simulink model "TTypeInverter_R2022a"  (R2022a)
settings: Solver=ode23t  StartTime=0.0  StopTime=0.2  RelTol=1e-3  EnableMultiTasking=on
values from neighbouring files (symbols this model uses):
  C_c = 30*10^-6    (= 3e-05)    [TTypeInverterVals.m]
  den = abs(G_pr_r_z.Denominator{1,1})    [TTypeInverterVals.m]
  den15 = abs(G_pr_r_15_z.Denominator{1,1})    [TTypeInverterVals.m]
  den21 = abs(G_pr_r_21_z.Denominator{1,1})    [TTypeInverterVals.m]
  den5 = abs(G_pr_r_5_z.Denominator{1,1})    [TTypeInverterVals.m]
  den7 = abs(G_pr_r_7_z.Denominator{1,1})    [TTypeInverterVals.m]
  f_o = 50    [TTypeInverterVals.m]
  G_diff_z = c2d(G_diff_s,Ts,opt)    [ControllerDesign.m]    (also in TTypeInverterVals.m = c2d(G_diff_s,Ts,'foh'))
  Kc = 2.5    [ControllerDesign.m]    (also in TTypeInverterVals.m)
  Klim = 5    [TTypeInverterVals.m]
  Kp = 1/mag/(10^(1.14/20))    [ControllerDesign.m]    (also in TTypeInverterVals.m = 0.9444)
  Kr = omega_c_o/2    (= 3141.59265359)    [ControllerDesign.m]    (also in TTypeInverterVals.m)
  N = 26    [Inductance.m]    (also in TTypeInverterVals.m = [0])
  num = abs(G_pr_r_z.Numerator{1,1})    [TTypeInverterVals.m]
  num15 = abs(G_pr_r_15_z.Numerator{1,1})    [TTypeInverterVals.m]
  num21 = abs(G_pr_r_21_z.Numerator{1,1})    [TTypeInverterVals.m]
  num5 = abs(G_pr_r_5_z.Numerator{1,1})    [TTypeInverterVals.m]
  num7 = abs(G_pr_r_7_z.Numerator{1,1})    [TTypeInverterVals.m]
  omega_o = fo*2*pi    (= 314.159265359)    [ControllerDesign.m]    (also in TTypeInverterVals.m)
  omega_w = 0.1*2*pi    (= 0.628318530718)    [ControllerDesign.m]    (also in TTypeInverterVals.m)
  pr_sat_val = ceil(3*io_nom)    [TTypeInverterVals.m]
  Q = eye(3)    [TTypeInverterVals.m]
  R = [R_iL 0 ... (first row only)    [TTypeInverterVals.m]
  R_l_20p = Vout^2/P_lin_20p    (= 10.58)    [TTypeInverterVals.m]
  R_l_3p = Vout/(P_max_3p/(Vout*3))    (= 2.116)    [TTypeInverterVals.m]
  R_l_80p = Vout^2/P_lin_80p    (= 2.645)    [TTypeInverterVals.m]
  R_l_nl = Vout^2/P_lin    (= 3.11176470588)    [TTypeInverterVals.m]
  R_l_nl_3p = Vout_3p^2/P_lin_3p    [TTypeInverterVals.m]
  R_Lc = 5.6e-3    (= 0.0056)    [TTypeInverterVals.m]
  R_nl_load = Uc^2/(0.66*S_tot)    (= 14.9121893939)    [TTypeInverterVals.m]
  R_nl_load_3p = Uc_3p^2/(0.66*S_tot_3p)    (= 4.97072979798)    [TTypeInverterVals.m]
  R_nl_s = 0.04*Vout^2/S_tot    (= 0.2645)    [TTypeInverterVals.m]
  R_nl_s_3p = 0.04*Vout_3p^2/S_tot_3p    [TTypeInverterVals.m]
  T_sw = 1/f_sw    (= 4.16666666667e-05)    [TTypeInverterVals.m]
  Tcomp = Ts/4    (= 2.60400009204e-06)    [TTypeInverterVals.m]
  Ts = 1/fs    (= 1.04166666667e-05)    [ControllerDesign.m]    (also in KalmanFilter.m = 2.08333333333e-05; TTypeInverterVals.m = 1.04160003681e-05)
  VDC = 800    [TTypeInverterVals.m]
  Vout_amp = Vout*sqrt(2)    [TTypeInverterVals.m]
undefined symbols (not defined in the file or in its folder): a0, a1, b0, b1, Discrete, G_ll_z, Ki, Kpc, KT, kv, Time, UKF_data
libraries: ee_lib x94, nesl_utility x48, fl_lib x39, dspstat3 x15, spsTriangleGeneratorLib x6, ctrlSharedLib x3, spsRMSLib x3, spsTHDLib x3
(part 3 of 5)

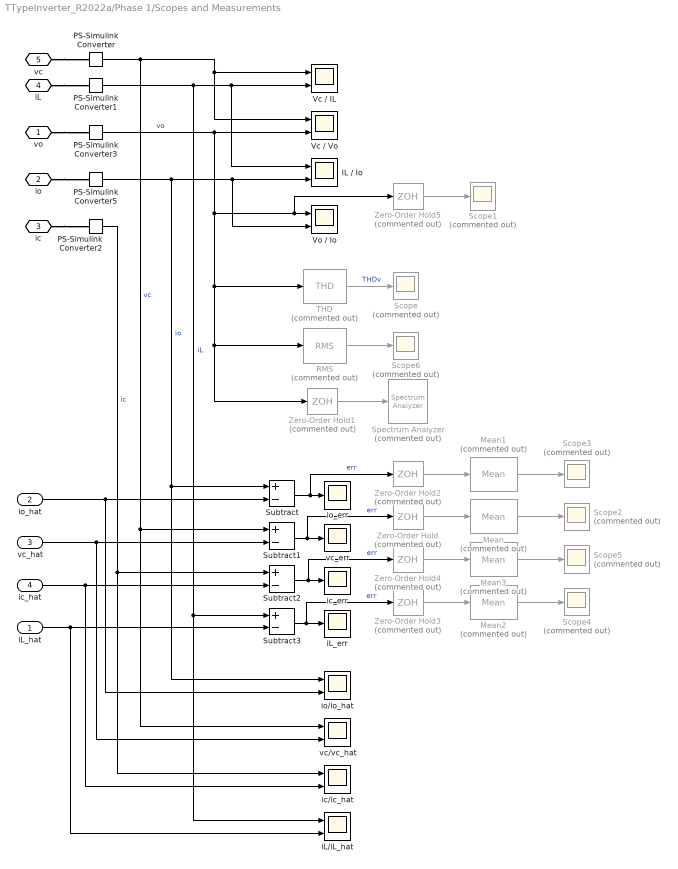
== system TTypeInverter_R2022a/Phase 1/Scopes and Measurements ==
  iL_hat : Inport
  io_hat : Inport  Port=2
  vc_hat : Inport  Port=3
  ic_hat : Inport  Port=4
  IL / Io : Scope  NumInputPorts=2
  Mean{,1..3} (4 alike) : dspstat3/Mean  Commented=on  run=on  InputProcessing=Columns as channels (frame based)  reset_popup=None  directionMode=Each column  dimension=1  roiEnable=off  roiType=Rectangles  roiPortion=Entire ROI  roiOutput=Individual statistics for each ROI  roiFlag=off  roundingMode=Floor  overflowMode=off  outputDataTypeStr=Inherit: Same as accumulator  outputMin=[]  outputMax=[]  outputLastDataTypeStr=Inherit: Same as accumulator
  PS-Simulink Converter{,1..3,5} (5 alike) : nesl_utility/PS-Simulink Converter  PhysicalDomain=network_engine_domain  SubClassName=ps_output  LeftPortType=input  RightPortType=output  PseudoPeriodic=off  Frequencies=[]  VectorFormat=inherit  Unit=inherit  AffineConversion=off
      settings: SourceProductBaseCode=SS,PW,VE
  RMS : spsRMSLib/RMS  Commented=on  TrueRMS=on  Freq=100  RMSInit=230  Ts=0
  Scope{,1..6} (7 alike) : Scope  Commented=on
  Spectrum Analyzer : SpectrumAnalyzer  Commented=on
  Subtract{,1..3} (4 alike) : Sum  Inputs=+-
  THD : spsTHDLib/THD  Commented=on  Freq=50  Ts=0
      settings: SourceProductBaseCode=PS
  Vc / IL : Scope  NumInputPorts=2
  Vc / Vo : Scope  NumInputPorts=2
  Vo / Io : Scope  NumInputPorts=2
  Zero-Order Hold{,2..4} (4 alike) : ZeroOrderHold  Commented=on  SampleTime=Ts/10
  Zero-Order Hold1 : ZeroOrderHold  Commented=on  SampleTime=1/100000
  Zero-Order Hold5 : ZeroOrderHold  Commented=on  SampleTime=T_sw/500
  iL/iL_hat : Scope  NumInputPorts=2
  iL_err : Scope
  ic/ic_hat : Scope  NumInputPorts=2
  ic_err : Scope
  io/io_hat : Scope  NumInputPorts=2
  io_err : Scope
  vc/vc_hat : Scope  NumInputPorts=2
  vc_err : Scope
  vo : PMIOPort  Side=Left
  io : PMIOPort  Port=2  Side=Left
  ic : PMIOPort  Port=3  Side=Left
  iL : PMIOPort  Port=4  Side=Left
  vc : PMIOPort  Port=5  Side=Left
  wires:
  PS-Simulink Converter1/1 -> iL/iL_hat/1, Subtract3/1, IL / Io/1, Vc / IL/2  "iL"
  PS-Simulink Converter/1 -> vc/vc_hat/1, Subtract1/1, Vc / Vo/1, Vc / IL/1  "vc"
  THD/1 -> Scope/1  "THDv"
  PS-Simulink Converter5/1 -> io/io_hat/1, Subtract/1, Vo / Io/2, IL / Io/2  "io"
  PS-Simulink Converter3/1 -> Vc / Vo/2, Zero-Order Hold5/1, Vo / Io/1, THD/1, RMS/1, Zero-Order Hold1/1  "vo"
  Zero-Order Hold1/1 -> Spectrum Analyzer/1
  io_hat/1 -> io/io_hat/2, Subtract/2
  Subtract/1 -> Zero-Order Hold2/1, io_err/1  "err"
  ic_hat/1 -> ic/ic_hat/2, Subtract2/2
  vc_hat/1 -> vc/vc_hat/2, Subtract1/2
  Subtract1/1 -> Zero-Order Hold/1, vc_err/1  "err"
  PS-Simulink Converter2/1 -> ic/ic_hat/1, Subtract2/1  "ic"
  Subtract2/1 -> Zero-Order Hold4/1, ic_err/1  "err"
  Mean/1 -> Scope2/1
  Zero-Order Hold/1 -> Mean/1
  Mean1/1 -> Scope3/1
  Zero-Order Hold2/1 -> Mean1/1
  iL_hat/1 -> iL/iL_hat/2, Subtract3/2
  Subtract3/1 -> Zero-Order Hold3/1, iL_err/1  "err"
  Mean2/1 -> Scope4/1
  Zero-Order Hold3/1 -> Mean2/1
  Mean3/1 -> Scope5/1
  Zero-Order Hold4/1 -> Mean3/1
  RMS/1 -> Scope6/1
  Zero-Order Hold5/1 -> Scope1/1
  connections:
  vc/RConn1 -- PS-Simulink Converter/LConn1
  iL/RConn1 -- PS-Simulink Converter1/LConn1
  vo/RConn1 -- PS-Simulink Converter3/LConn1
  io/RConn1 -- PS-Simulink Converter5/LConn1
  ic/RConn1 -- PS-Simulink Converter2/LConn1

== system TTypeInverter_R2022a/Phase 2/Controllers ==
  note: Voltage feedforward
  note: Current feedforward
  iL : Inport
  io_hat : Inport  Port=2
  vc : Inport  Port=3
  ic_hat : Inport  Port=4
  Current Controller : Subsystem
  Error Scope : Scope  NumInputPorts=2
  Gain : Gain  Gain=2/VDC
  Gain1 : Gain  Gain=R_Lc
  Reference Scope : Scope  NumInputPorts=2
  Saturation : Saturate  UpperLimit=VDC/2  LowerLimit=-VDC/2
  Sine Wave : Sin  Amplitude=Vout_amp  Frequency=f_o*2*pi  Phase=120*pi/180  SampleTime=Ts
  Sum : Sum  Inputs=|+-
  Sum1 : Sum  Inputs=++|
  Sum2 : Sum  Inputs=+++
  Sum3 : Sum  Inputs=-+|
  Transport Delay : TransportDelay  DelayTime=Tcomp
  Voltage Controller : Subsystem
  m : Outport
  vi_ref : Outport  Port=2
  wires:
  Transport Delay/1 -> m/1
  Voltage Controller/1(Out) -> Sum1/2, Reference Scope/2  "iL_ref"
  Sum/1 -> Error Scope/2, Voltage Controller/1(In)  "e_vc"
  Gain/1 -> Transport Delay/1  "m"
  vc/1 -> Sum/2, Sum2/3  "vc"
  iL/1 -> Sum3/1, Current Controller/1(iL), Gain1/1  "iL"
  Sum2/1 -> Saturation/1
  Gain1/1 -> Sum2/1  "vRLc"
  Sine Wave/1 -> Sum/1  "vc_ref"
  Sum3/1 -> Error Scope/1, Current Controller/2(In)  "e_iL"
  Sum1/1 -> Sum3/2
  io_hat/1 -> Sum1/1  "io"
  Current Controller/1(Out) -> Sum2/2
  Saturation/1 -> vi_ref/1, Reference Scope/1, Gain/1  "vi_ref"

== system TTypeInverter_R2022a/Phase 2/Inverter ==
  Capacitor : ee_lib/Passive/Capacitor  cap_option=0  c=30e-6 F  Cvec=[1e-05, 1e-06] F  Vvec=[0, 10] V  CV_table_symmetry=1  f_vec=[1, 10] kHz  DFext_vec=[.8, 1.2]  enable_C_tol=0  C_tol=5  tol_distribution=1  nSigma=4  r=1e-6 Ohm  g=0 1/Ohm  averaging_period=0 s  enable_operating_limits=0  operating_limit_action=2  max_working_voltage_range=[-25, 25] V  power_rating=1 W  enable_faults=0  fault_action=1  Cscale_faulted=100  R_faulted=1e-3 Ohm  G_faulted=0 1/Ohm  tau_fault=1e-3 s  enable_temporal_fault=0  t_fault=1 s  enable_behavioral_fault=0  max_permissible_voltage_range=[-100, 100] V  t_fail_on_voltage=1 s  i_specify=off  i_priority=None  i=0 A  i_nominal_specify=off  i_nominal_unit=A  i_nominal_value=1  v_specify=off  v_priority=None  v=0 V  v_nominal_specify=off  v_nominal_unit=V  v_nominal_value=1  vc_specify=off  vc_priority=High  vc=0 V  vc_nominal_specify=off  vc_nominal_unit=V  vc_nominal_value=1
  Capacitor1 : ee_lib/Passive/Capacitor  cap_option=0  c=30e-6 F  Cvec=[1e-05, 1e-06] F  Vvec=[0, 10] V  CV_table_symmetry=1  f_vec=[1, 10] kHz  DFext_vec=[.8, 1.2]  enable_C_tol=0  C_tol=5  tol_distribution=1  nSigma=4  r=1e-6 Ohm  g=0 1/Ohm  averaging_period=0 s  enable_operating_limits=0  operating_limit_action=2  max_working_voltage_range=[-25, 25] V  power_rating=1 W  enable_faults=0  fault_action=1  Cscale_faulted=100  R_faulted=1e-3 Ohm  G_faulted=0 1/Ohm  tau_fault=1e-3 s  enable_temporal_fault=0  t_fault=1 s  enable_behavioral_fault=0  max_permissible_voltage_range=[-100, 100] V  t_fail_on_voltage=1 s  i_specify=off  i_priority=None  i=0 A  i_nominal_specify=off  i_nominal_unit=A  i_nominal_value=1  v_specify=off  v_priority=None  v=0 V  v_nominal_specify=off  v_nominal_unit=V  v_nominal_value=1  vc_specify=off  vc_priority=High  vc=0 V  vc_nominal_specify=off  vc_nominal_unit=V  vc_nominal_value=1
  Gate Driver{1..4} (4 alike) : ee_lib/Semiconductors & Converters/Gate Driver  uHighValue=0.7  uLowValue=0.3  vHigh=15 V  vLow=0 V  tHigh=T_on ns  tLow=T_off ns  parameterization=1  rHigh=R_on Ohm  rLow=R_off Ohm  tRise=20 ns  tFall=20 ns  cLoad=10 nF  enable_faults=0  t_fault=1 s  fault_type=1  ZonTime_specify=off  ZonTime_priority=None  ZonTime=0 s  ZoffTime_specify=off  ZoffTime_priority=None  ZoffTime=0 s  uHigh=2.0 V  uLow=0.8 V
      settings: SourceProductBaseCode=PS  InternalSimscapePortConfiguration="{\"Bottom\":[],\"Left\":[{\"id\":\"u\",\"label\":\"u\",\"type\":\"input\"}],\"Right\":[{\"id\":\"G\",\"label\":\"G\",\"type\":\"foundation.electrical.electrical\"},{\"id\":\"S\",\"label\":\"S\",\"type\":\"foundation.electrical.electrical\"}],\"Top\":[]}"
  S{1..4} (4 alike) : ee_lib/Semiconductors & Converters/IGBT (Ideal, Switching)  Vf=V_ft V  Ron=R_ont Ohm  Goff=1e-5 1/Ohm  Vth=6 V  diode_param=2  diode_Vf=V_fd V  diode_Ron=R_ond Ohm  diode_Goff=1e-5 1/Ohm  diode_C=50e-9 F  diode_iRM=-235 A  diode_iF=300 A  diode_idot=-50 A/us  diode_trr_param=ee.enum.converters.diodeReverseParam.trr_factor  diode_trr_factor=3  diode_trr=15 us  diode_Qrr=1500 s*uA  thermal_loss_option=ee.enum.converters.thermalLossOption.constantvalues  Von_data=[0, .1, .6, .8, 1, 1.3, 1.6, 2, 2.4; 0, .1, .7, 1, 1.2, 1.5, 1.9, 2.4, 2.8] V  Tj=[298.15, 398.15] K  Iout_data=[0, .1, 1, 5, 10, 20, 40, 70, 100] A  Eon_data=[0, .0024, .024, .12, .2, .48, 1.04, 2.16, 3.24; 0, .003, .03, .15, .25, .6, 1.3, 2.7, 4.05] * 1e-3 J  Eoff_data=[0, .0007, .0066, .033, .066, .17, .33, .83, 1.5; 0, .001, .01, .05, .1, .25, .5, 1.2, 2.2] * 1e-3 J  Tj_loss=[298.15, 398.15] K  Iout_data_loss=[0, .1, 1, 5, 10, 20, 40, 70, 100] A  Eon_scalar=22.86e-3 J  Eoff_scalar=17.14e-3 J  Voff=300 V  Iout_scalar=600 A  diodeModelType=ee.enum.converters.diodeModelType.pwl  diodeTableType=ee.enum.diode.tableType.IfMat  diode_IfMat=[.07, .12, .19, 1.75, 4.24, 7.32, 11.2; .16, .3, .72, 2.14, 4.02, 6.35, 9.12] A  diode_VfMat=[.9, 1.15, 1.25, 1.5, 1.75, 2.17, 2.6, 2.85; .58, .68, .75, 1.1, 1.38, 1.77, 2.27, 2.7] V  diode_TjVec=[25, 125] degC  diode_VfVec=[.5, .7, .9, 1.3, 1.7, 2.1, 2.5] V  diode_IfVec=[.1, .2, .5, 1, 2, 4, 7, 10] A  diode_Vr=-600 V  diode_Ls=150 nH  diode_Erec=0.03 J  thermal_network_parameterization=ee.enum.thermalNetworkTopology.external  Rth=[.08, .5] K/W  Rth_Cauer=[.08, .1, .5] K/W  Rth_Foster=[.08, .14, .22, .16] K/W  thermal_mass_parameterization=ee.enum.thermalNetwork.timeconstant  thermal_mass=[.01, .5] J/K  thermal_mass_Cauer=[.01, .1, .5] J/K  thermal_mass_Foster=[.001, .005, .05, .5] J/K  thermal_time_constant=[.001, .2] s  thermal_time_constant_Cauer=[.001, .1, .2] s  thermal_time_constant_Foster=[7e-05, .0007, .01, .08] s  thermal_mass_initial_temperatures=[25, 25] degC  thermal_mass_initial_temperatures_Cauer=[25, 25, 25] degC  junction_thermal_mass=0.01 J/K  steadyState_Foster=simscape.enum.onoff.on  Tvec_initial_Foster=[25, 25, 25, 25] degC  no_thermal_network=0  junction_temperature_specify=off  junction_temperature_priority=None  junction_temperature=25 degC  junction_temperature_nominal_specify=off  junction_temperature_nominal_unit=degC  junction_temperature_nominal_value=1  vT_specify=off  vT_priority=None  vT=0 V  vT_nominal_specify=off  vT_nominal_unit=V  vT_nominal_value=1  Qj_specify=off  Qj_priority=None  Qj=0 W  Qj_nominal_specify=off  Qj_nominal_unit=W  Qj_nominal_value=1
      settings: InternalSimscapePortConfiguration="{\"Bottom\":[],\"Left\":[{\"id\":\"G\",\"label\":\"\",\"type\":\"foundation.electrical.electrical\"}],\"Right\":[{\"id\":\"C\",\"label\":\"\",\"type\":\"foundation.electrical.electrical\"},{\"id\":\"E\",\"label\":\"\",\"type\":\"foundation.electrical.electrical\"}],\"Top\":[]}"
  vi : PMIOPort  Side=Right
  Q1 : PMIOPort  Port=2  Side=Left
  Q2 : PMIOPort  Port=3  Side=Left
  Q3 : PMIOPort  Port=4  Side=Left
  Q4 : PMIOPort  Port=5  Side=Left
  DC+ : PMIOPort  Port=6  Side=Left
  DC- : PMIOPort  Port=7  Side=Left
  GND : PMIOPort  Port=8  Side=Left
  connections:
  Capacitor1/RConn1 -- DC-/RConn1 -- Gate Driver3/RConn2 -- S4/RConn2
  S3/RConn1 -- vi/RConn1 -- S1/RConn2 -- Gate Driver4/RConn2 -- S4/RConn1
  GND/RConn1 -- Capacitor1/LConn1 -- Capacitor/RConn1 -- S2/RConn1
  Capacitor/LConn1 -- DC+/RConn1 -- S1/RConn1
  Gate Driver4/LConn1 -- Q1/RConn1
  Q3/RConn1 -- Gate Driver2/LConn1
  Gate Driver3/LConn1 -- Q4/RConn1
  S3/RConn2 -- Gate Driver1/RConn2 -- Gate Driver2/RConn2 -- S2/RConn2
  S1/LConn1 -- Gate Driver4/RConn1
  S4/LConn1 -- Gate Driver3/RConn1
  Gate Driver1/LConn1 -- Q2/RConn1
  S2/LConn1 -- Gate Driver1/RConn1
  S3/LConn1 -- Gate Driver2/RConn1

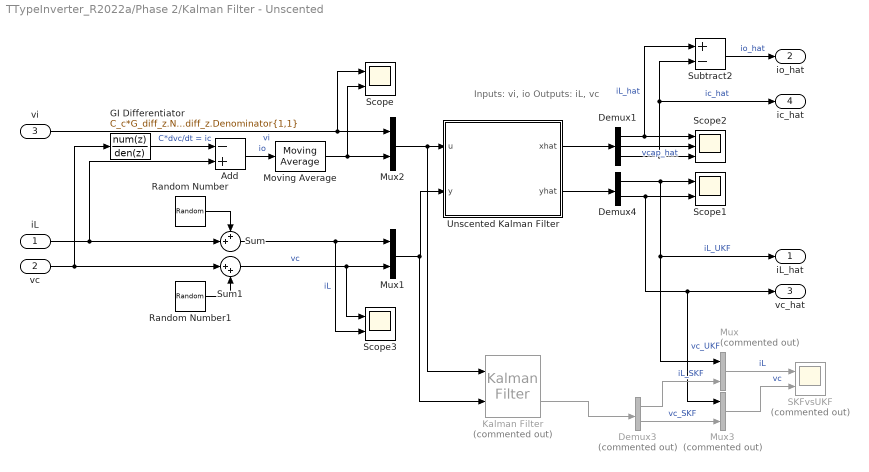
== system TTypeInverter_R2022a/Phase 2/Kalman Filter - Unscented ==
  note: Inputs: vi, io
      | Outputs: iL, vc
  iL : Inport
  vc : Inport  Port=2
  vi : Inport  Port=3
  Add : Sum  Inputs=-+
  Demux1 : Demux  Outputs=3
  Demux3 : Demux  Commented=on  Outputs=2
  Demux4 : Demux  Outputs=2
  GI Differentiator : DiscreteTransferFcn  Numerator=C_c*G_diff_z.Numerator{1,1}  Denominator=G_diff_z.Denominator{1,1}  SampleTime=Ts
  Kalman Filter : ctrlSharedLib/Kalman Filter  Commented=on  TimeDomain=Discrete-Time  UseCurrentEstimator=on  ModelSource=LTI State-Space Variable  ModelSourceVariable=lcl_sys_z  A=0.95  B=1  C=1  D=0  NumberOfStates=1  NumberOfInputs=1  NumberOfOutputs=1  InitialEstimateSource=Dialog  X0=0  P0=10  UseK=off  UseGH=off  NumberOfProcessNoiseInputs=1  G=1  TimeInvariantG=on  H=0  TimeInvariantH=on  Q=Q(1)  TimeInvariantQ=on  R=R  TimeInvariantR=on  N=N  TimeInvariantN=on  AddInputPort=on  AddEnablePort=off  OutputEstimatedY=on  OutputP=off  Ts=-1
  Moving Average : dspstat3/Moving Average  Method=Sliding window  ForgettingFactorPort=off  SpecifyWindowLength=on  WindowLength=4  ForgettingFactor=0.9  SimulateUsing=Code generation
  Mux : Mux  Commented=on  Inputs=2
  Mux1 : Mux  Inputs=2
  Mux2 : Mux  Inputs=2
  Mux3 : Mux  Commented=on  Inputs=2
  Random Number : RandomNumber  Variance=R(1,1)  SampleTime=Ts
  Random Number1 : RandomNumber  Variance=R(2,2)  SampleTime=Ts
  SKFvsUKF : Scope  Commented=on  NumInputPorts=2
  Scope : Scope  NumInputPorts=2
  Scope1 : Scope  NumInputPorts=2
  Scope2 : Scope  NumInputPorts=3
  Scope3 : Scope  NumInputPorts=2
  Subtract2 : Sum  Inputs=+-
  Sum : Sum  Inputs=++|
  Sum1 : Sum  Inputs=|++
  Unscented Kalman Filter : Subsystem
  iL_hat : Outport
  io_hat : Outport  Port=2
  vc_hat : Outport  Port=3
  ic_hat : Outport  Port=4
  wires:
  Demux4/1 -> Mux/1, iL_hat/1, Scope1/1  "iL_UKF"
  Demux1/2 -> Scope2/2  "vcap_hat"
  Demux1/3 -> ic_hat/1, Subtract2/2, Scope2/3  "ic_hat"
  Demux1/1 -> Subtract2/1, Scope2/1  "iL_hat"
  Mux1/1 -> Kalman Filter/2, Unscented Kalman Filter/2(y)
  GI Differentiator/1 -> Add/1  "C*dvc/dt = ic"
  vi/1 -> Scope/1, Mux2/1  "vi"
  Demux4/2 -> Scope1/2, Mux3/1, vc_hat/1  "vc_UKF"
  Unscented Kalman Filter/2(yhat) -> Demux4/1
  vc/1 -> Sum1/1, GI Differentiator/1
  Unscented Kalman Filter/1(xhat) -> Demux1/1
  iL/1 -> Sum/2, Add/2
  Sum/1 -> Scope3/2, Mux1/1  "iL"
  Sum1/1 -> Scope3/1, Mux1/2  "vc"
  Random Number/1 -> Sum/1
  Random Number1/1 -> Sum1/2
  Mux2/1 -> Kalman Filter/1, Unscented Kalman Filter/1(u)
  Subtract2/1 -> io_hat/1  "io_hat"
  Add/1 -> Moving Average/1  "io"
  Moving Average/1 -> Mux2/2, Scope/2
  Kalman Filter/2 -> Demux3/1
  Mux/1 -> SKFvsUKF/1  "iL"
  Demux3/1 -> Mux/2  "iL_SKF"
  Mux3/1 -> SKFvsUKF/2  "vc"
  Demux3/2 -> Mux3/2  "vc_SKF"

== system TTypeInverter_R2022a/Phase 2/Output Filter ==
  Cc : ee_lib/Passive/Capacitor  cap_option=0  c=C_c F  Cvec=[1e-05, 1e-06] F  Vvec=[0, 10] V  CV_table_symmetry=1  f_vec=[1, 10] kHz  DFext_vec=[.8, 1.2]  enable_C_tol=0  C_tol=5  tol_distribution=1  nSigma=4  r=R_Cc Ohm  g=0 1/Ohm  averaging_period=0 s  enable_operating_limits=0  operating_limit_action=2  max_working_voltage_range=[-25, 25] V  power_rating=1 W  enable_faults=0  fault_action=1  Cscale_faulted=100  R_faulted=1e-3 Ohm  G_faulted=0 1/Ohm  tau_fault=1e-3 s  enable_temporal_fault=0  t_fault=1 s  enable_behavioral_fault=0  max_permissible_voltage_range=[-100, 100] V  t_fail_on_voltage=1 s  i_specify=off  i_priority=None  i=0 A  i_nominal_specify=off  i_nominal_unit=A  i_nominal_value=1  v_specify=off  v_priority=None  v=0 V  v_nominal_specify=off  v_nominal_unit=V  v_nominal_value=1  vc_specify=off  vc_priority=High  vc=280 V  vc_nominal_specify=off  vc_nominal_unit=V  vc_nominal_value=1
  Cr : ee_lib/Passive/Capacitor  cap_option=0  c=C_r F  Cvec=[1e-05, 1e-06] F  Vvec=[0, 10] V  CV_table_symmetry=1  f_vec=[1, 10] kHz  DFext_vec=[.8, 1.2]  enable_C_tol=0  C_tol=5  tol_distribution=1  nSigma=4  r=R_Cr Ohm  g=0 1/Ohm  averaging_period=0 s  enable_operating_limits=0  operating_limit_action=2  max_working_voltage_range=[-25, 25] V  power_rating=1 W  enable_faults=0  fault_action=1  Cscale_faulted=100  R_faulted=1e-3 Ohm  G_faulted=0 1/Ohm  tau_fault=1e-3 s  enable_temporal_fault=0  t_fault=1 s  enable_behavioral_fault=0  max_permissible_voltage_range=[-100, 100] V  t_fail_on_voltage=1 s  i_specify=off  i_priority=None  i=0 A  i_nominal_specify=off  i_nominal_unit=A  i_nominal_value=1  v_specify=off  v_priority=None  v=0 V  v_nominal_specify=off  v_nominal_unit=V  v_nominal_value=1  vc_specify=off  vc_priority=High  vc=0 V  vc_nominal_specify=off  vc_nominal_unit=V  vc_nominal_value=1
  Current Sensor : fl_lib/Electrical/Electrical Sensors/Current Sensor
      settings: SourceProductBaseCode=PW,SS,VE
  Current Sensor2 : fl_lib/Electrical/Electrical Sensors/Current Sensor
      settings: SourceProductBaseCode=PW,SS,VE
  Electrical Reference1 : fl_lib/Electrical/Electrical Elements/Electrical Reference
      settings: SourceProductBaseCode=PW,SS,VE
  Lc : ee_lib/Passive/Inductor  l=L_c H  enable_L_tol=0  L_tol=20  tol_distribution=1  nSigma=4  r=R_Lc Ohm  g=1e-9 1/Ohm  enable_operating_limits=0  operating_limit_action=2  max_working_current=1 A  power_rating=1 W  enable_faults=0  fault_action=1  lambdaPercent=50  k_faulted=0.9999  turnsShort=0  openCct=0  groundShort=0  groundShortG=0 1/Ohm  tau_fault=1e-3 s  enable_temporal_fault=0  t_fault=1 s  enable_behavioral_fault=0  max_permissible_voltage=100 V  n_fail_on_voltage=1  max_permissible_current=1 A  t_fail_on_current=1 s  i_L_specify=off  i_L_priority=High  i_L=0 A  i_L_nominal_specify=off  i_L_nominal_unit=A  i_L_nominal_value=1
  "Lc (Nonlinear, phi-I)" : ee_lib/Passive/Nonlinear Inductor  parameterization_option=3  Nw=N_Lc  L=2e-4 H  L_sat=1e-4 H  current_data=Lc_nonlin_i A  magnetic_flux_data=Lc_nonlin_phi Wb  H_data=[0, 200, 400, 600, 800, 1000] A/m  B_data=[0, .81, 1.25, 1.42, 1.48, 1.49] T  magnetic_flux_sat=1.3e-05 Wb  length_effective=0.032 m  area_effective=1.6e-5 m^2  dBdH0=0.005 T*m/A  B1=1.49 T  H1=1000 A/m  c=0.1  K=200 A/m  alpha=1e-4  averaging_period=0 s  G_parasitic=1e-9 1/Ohm  interpolation_option=1  x0_option=1  i_L0=0 A  phi0=0 Wb  B0=0 T  H0=0 A/m
      settings: SourceProductBaseCode=PS  InternalSimscapePortConfiguration="{\"Bottom\":[],\"Left\":[{\"id\":\"p\",\"label\":\"+\",\"type\":\"foundation.electrical.electrical\"}],\"Right\":[{\"id\":\"n\",\"label\":\"-\",\"type\":\"foundation.electrical.electrical\"}],\"Top\":[]}"
  Lg : ee_lib/Passive/Inductor  l=L_g H  enable_L_tol=0  L_tol=20  tol_distribution=1  nSigma=4  r=R_Lg Ohm  g=1e-9 1/Ohm  enable_operating_limits=0  operating_limit_action=2  max_working_current=1 A  power_rating=1 W  enable_faults=0  fault_action=1  lambdaPercent=50  k_faulted=0.9999  turnsShort=0  openCct=0  groundShort=0  groundShortG=0 1/Ohm  tau_fault=1e-3 s  enable_temporal_fault=0  t_fault=1 s  enable_behavioral_fault=0  max_permissible_voltage=100 V  n_fail_on_voltage=1  max_permissible_current=1 A  t_fail_on_current=1 s  i_L_specify=off  i_L_priority=High  i_L=0 A  i_L_nominal_specify=off  i_L_nominal_unit=A  i_L_nominal_value=1
  Lr : ee_lib/Passive/Inductor  l=L_r H  enable_L_tol=0  L_tol=20  tol_distribution=1  nSigma=4  r=R_Lr Ohm  g=1e-9 1/Ohm  enable_operating_limits=0  operating_limit_action=2  max_working_current=1 A  power_rating=1 W  enable_faults=0  fault_action=1  lambdaPercent=50  k_faulted=0.9999  turnsShort=0  openCct=0  groundShort=0  groundShortG=0 1/Ohm  tau_fault=1e-3 s  enable_temporal_fault=0  t_fault=1 s  enable_behavioral_fault=0  max_permissible_voltage=100 V  n_fail_on_voltage=1  max_permissible_current=1 A  t_fail_on_current=1 s  i_L_specify=off  i_L_priority=High  i_L=0 A  i_L_nominal_specify=off  i_L_nominal_unit=A  i_L_nominal_value=1
  RLc : fl_lib/Electrical/Electrical Elements/Resistor  R=R_Lc Ohm  i_specify=off  i_priority=None  i=0 A  i_nominal_specify=off  i_nominal_unit=A  i_nominal_value=1  v_specify=off  v_priority=None  v=0 V  v_nominal_specify=off  v_nominal_unit=V  v_nominal_value=1
      settings: SourceProductBaseCode=PW,SS,VE
  Voltage Sensor : fl_lib/Electrical/Electrical Sensors/Voltage Sensor
      settings: SourceProductBaseCode=PW,SS,VE
  vi : PMIOPort  Side=Left
  vo : PMIOPort  Port=2  Side=Right
  GND : PMIOPort  Port=3  Side=Right
  ic : PMIOPort  Port=4  Side=Right
  vc : PMIOPort  Port=5  Side=Right
  iL : PMIOPort  Port=6  Side=Right
  connections:
  Lr/LConn1 -- Cr/RConn1
  Voltage Sensor/RConn1 -- vc/RConn1
  Current Sensor/LConn1 -- vi/RConn1
  Electrical Reference1/LConn1 -- Voltage Sensor/RConn2 -- Cc/RConn1 -- Lr/RConn1 -- GND/RConn1
  Lg/RConn1 -- vo/RConn1
  Voltage Sensor/LConn1 -- Current Sensor2/LConn1 -- Lg/LConn1 -- Cr/LConn1 -- RLc/RConn1
  "Lc (Nonlinear, phi-I)"/LConn1 -- Current Sensor/RConn2
  Current Sensor/RConn1 -- iL/RConn1
  Current Sensor2/RConn2 -- Cc/LConn1
  Current Sensor2/RConn1 -- ic/RConn1
  "Lc (Nonlinear, phi-I)"/RConn1 -- RLc/LConn1

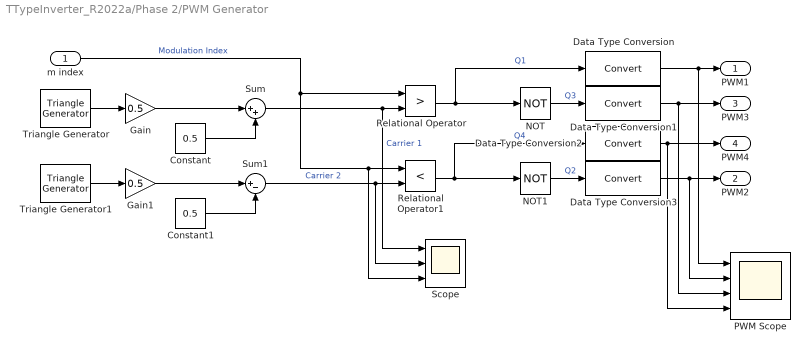
== system TTypeInverter_R2022a/Phase 2/PWM Generator ==
  m index : Inport
  Constant : Constant  Value=0.5
  Constant1 : Constant  Value=0.5
  Data Type Conversion{,1..3} (4 alike) : DataTypeConversion  SaturateOnIntegerOverflow=off  RndMeth=Floor
  Gain : Gain  Gain=0.5
  Gain1 : Gain  Gain=0.5
  NOT : Logic  Operator=NOT  IconShape=distinctive  AllPortsSameDT=off  OutDataTypeStr=boolean
  NOT1 : Logic  Operator=NOT  IconShape=distinctive  AllPortsSameDT=off  OutDataTypeStr=boolean
  PWM Scope : Scope  NumInputPorts=4
  Relational Operator : RelationalOperator  Operator=>  OutDataTypeStr=boolean  RndMeth=Simplest  InputSameDT=off
  Relational Operator1 : RelationalOperator  Operator=<  OutDataTypeStr=boolean  RndMeth=Simplest  InputSameDT=off
  Scope : Scope  NumInputPorts=3
  Sum : Sum  Inputs=|++
  Sum1 : Sum  Inputs=|+-
  Triangle Generator : spsTriangleGeneratorLib/Triangle Generator  Freq=f_sw  Phase=0  Ts=0
  Triangle Generator1 : spsTriangleGeneratorLib/Triangle Generator  Freq=f_sw  Phase=0  Ts=0
  PWM1 : Outport
  PWM2 : Outport  Port=2
  PWM3 : Outport  Port=3
  PWM4 : Outport  Port=4
  wires:
  Relational Operator1/1 -> NOT1/1, Data Type Conversion2/1  "Q4"
  Data Type Conversion3/1 -> PWM2/1, PWM Scope/2
  Constant/1 -> Sum/2
  Gain/1 -> Sum/1
  NOT1/1 -> Data Type Conversion3/1  "Q2"
  NOT/1 -> Data Type Conversion1/1  "Q3"
  m index/1 -> Scope/3, Relational Operator1/1, Relational Operator/1  "Modulation Index"
  Data Type Conversion2/1 -> PWM4/1, PWM Scope/4
  Data Type Conversion1/1 -> PWM3/1, PWM Scope/3
  Triangle Generator1/1 -> Gain1/1
  Relational Operator/1 -> Data Type Conversion/1, NOT/1  "Q1"
  Data Type Conversion/1 -> PWM1/1, PWM Scope/1
  Triangle Generator/1 -> Gain/1
  Sum1/1 -> Scope/2, Relational Operator1/2  "Carrier 2"
  Sum/1 -> Scope/1, Relational Operator/2  "Carrier 1"
  Constant1/1 -> Sum1/2
  Gain1/1 -> Sum1/1

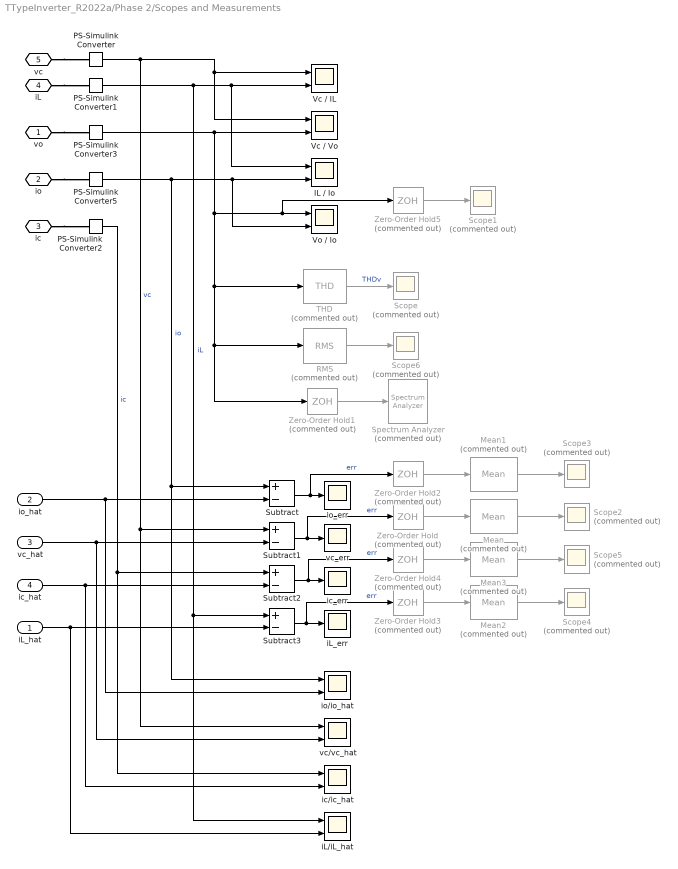
== system TTypeInverter_R2022a/Phase 2/Scopes and Measurements ==
  iL_hat : Inport
  io_hat : Inport  Port=2
  vc_hat : Inport  Port=3
  ic_hat : Inport  Port=4
  IL / Io : Scope  NumInputPorts=2
  Mean{,1..3} (4 alike) : dspstat3/Mean  Commented=on  run=on  InputProcessing=Columns as channels (frame based)  reset_popup=None  directionMode=Each column  dimension=1  roiEnable=off  roiType=Rectangles  roiPortion=Entire ROI  roiOutput=Individual statistics for each ROI  roiFlag=off  roundingMode=Floor  overflowMode=off  outputDataTypeStr=Inherit: Same as accumulator  outputMin=[]  outputMax=[]  outputLastDataTypeStr=Inherit: Same as accumulator
  PS-Simulink Converter{,1..3,5} (5 alike) : nesl_utility/PS-Simulink Converter  PhysicalDomain=network_engine_domain  SubClassName=ps_output  LeftPortType=input  RightPortType=output  PseudoPeriodic=off  Frequencies=[]  VectorFormat=inherit  Unit=inherit  AffineConversion=off
      settings: SourceProductBaseCode=SS,PW,VE
  RMS : spsRMSLib/RMS  Commented=on  TrueRMS=on  Freq=100  RMSInit=230  Ts=0
  Scope{,1..6} (7 alike) : Scope  Commented=on
  Spectrum Analyzer : SpectrumAnalyzer  Commented=on
  Subtract{,1..3} (4 alike) : Sum  Inputs=+-
  THD : spsTHDLib/THD  Commented=on  Freq=50  Ts=0
      settings: SourceProductBaseCode=PS
  Vc / IL : Scope  NumInputPorts=2
  Vc / Vo : Scope  NumInputPorts=2
  Vo / Io : Scope  NumInputPorts=2
  Zero-Order Hold{,2..4} (4 alike) : ZeroOrderHold  Commented=on  SampleTime=Ts/10
  Zero-Order Hold1 : ZeroOrderHold  Commented=on  SampleTime=1/100000
  Zero-Order Hold5 : ZeroOrderHold  Commented=on  SampleTime=T_sw/500
  iL/iL_hat : Scope  NumInputPorts=2
  iL_err : Scope
  ic/ic_hat : Scope  NumInputPorts=2
  ic_err : Scope
  io/io_hat : Scope  NumInputPorts=2
  io_err : Scope
  vc/vc_hat : Scope  NumInputPorts=2
  vc_err : Scope
  vo : PMIOPort  Side=Left
  io : PMIOPort  Port=2  Side=Left
  ic : PMIOPort  Port=3  Side=Left
  iL : PMIOPort  Port=4  Side=Left
  vc : PMIOPort  Port=5  Side=Left
  wires:
  PS-Simulink Converter1/1 -> iL/iL_hat/1, Subtract3/1, IL / Io/1, Vc / IL/2  "iL"
  PS-Simulink Converter/1 -> vc/vc_hat/1, Subtract1/1, Vc / Vo/1, Vc / IL/1  "vc"
  THD/1 -> Scope/1  "THDv"
  PS-Simulink Converter5/1 -> io/io_hat/1, Subtract/1, Vo / Io/2, IL / Io/2  "io"
  Zero-Order Hold1/1 -> Spectrum Analyzer/1
  io_hat/1 -> io/io_hat/2, Subtract/2
  Subtract/1 -> Zero-Order Hold2/1, io_err/1  "err"
  ic_hat/1 -> ic/ic_hat/2, Subtract2/2
  vc_hat/1 -> vc/vc_hat/2, Subtract1/2
  Subtract1/1 -> Zero-Order Hold/1, vc_err/1  "err"
  PS-Simulink Converter2/1 -> ic/ic_hat/1, Subtract2/1  "ic"
  Subtract2/1 -> Zero-Order Hold4/1, ic_err/1  "err"
  Mean/1 -> Scope2/1
  Zero-Order Hold/1 -> Mean/1
  Mean1/1 -> Scope3/1
  Zero-Order Hold2/1 -> Mean1/1
  iL_hat/1 -> iL/iL_hat/2, Subtract3/2
  Subtract3/1 -> Zero-Order Hold3/1, iL_err/1  "err"
  Mean2/1 -> Scope4/1
  Zero-Order Hold3/1 -> Mean2/1
  Mean3/1 -> Scope5/1
  Zero-Order Hold4/1 -> Mean3/1
  RMS/1 -> Scope6/1
  PS-Simulink Converter3/1 -> Vc / Vo/2, Zero-Order Hold5/1, Vo / Io/1, THD/1, RMS/1, Zero-Order Hold1/1
  Zero-Order Hold5/1 -> Scope1/1
  connections:
  vc/RConn1 -- PS-Simulink Converter/LConn1
  iL/RConn1 -- PS-Simulink Converter1/LConn1
  vo/RConn1 -- PS-Simulink Converter3/LConn1
  io/RConn1 -- PS-Simulink Converter5/LConn1
  ic/RConn1 -- PS-Simulink Converter2/LConn1

== system TTypeInverter_R2022a/Phase 3/Controllers ==
  note: Voltage feedforward
  note: Current feedforward
  iL : Inport
  io_hat : Inport  Port=2
  vc : Inport  Port=3
  ic_hat : Inport  Port=4
  Current Controller : Subsystem
  Error Scope : Scope  NumInputPorts=2
  Gain : Gain  Gain=2/VDC
  Gain1 : Gain  Gain=R_Lc
  Reference Scope : Scope  NumInputPorts=2
  Saturation : Saturate  UpperLimit=VDC/2  LowerLimit=-VDC/2
  Sine Wave : Sin  Amplitude=Vout_amp  Frequency=f_o*2*pi  Phase=240*pi/180  SampleTime=Ts
  Sum : Sum  Inputs=|+-
  Sum1 : Sum  Inputs=++|
  Sum2 : Sum  Inputs=+++
  Sum3 : Sum  Inputs=-+|
  Transport Delay : TransportDelay  DelayTime=Tcomp
  Voltage Controller : Subsystem
  m : Outport
  vi_ref : Outport  Port=2
  wires:
  Transport Delay/1 -> m/1
  Voltage Controller/1(Out) -> Sum1/2, Reference Scope/2  "iL_ref"
  Sum/1 -> Error Scope/2, Voltage Controller/1(In)  "e_vc"
  Gain/1 -> Transport Delay/1  "m"
  vc/1 -> Sum/2, Sum2/3  "vc"
  iL/1 -> Sum3/1, Current Controller/1(iL), Gain1/1  "iL"
  Sum2/1 -> Saturation/1
  Gain1/1 -> Sum2/1  "vRLc"
  Sine Wave/1 -> Sum/1  "vc_ref"
  Sum3/1 -> Error Scope/1, Current Controller/2(In)  "e_iL"
  Sum1/1 -> Sum3/2
  io_hat/1 -> Sum1/1  "io"
  Current Controller/1(Out) -> Sum2/2
  Saturation/1 -> vi_ref/1, Reference Scope/1, Gain/1  "vi_ref"

== system TTypeInverter_R2022a/Phase 3/Inverter ==
  Capacitor : ee_lib/Passive/Capacitor  cap_option=0  c=30e-6 F  Cvec=[1e-05, 1e-06] F  Vvec=[0, 10] V  CV_table_symmetry=1  f_vec=[1, 10] kHz  DFext_vec=[.8, 1.2]  enable_C_tol=0  C_tol=5  tol_distribution=1  nSigma=4  r=1e-6 Ohm  g=0 1/Ohm  averaging_period=0 s  enable_operating_limits=0  operating_limit_action=2  max_working_voltage_range=[-25, 25] V  power_rating=1 W  enable_faults=0  fault_action=1  Cscale_faulted=100  R_faulted=1e-3 Ohm  G_faulted=0 1/Ohm  tau_fault=1e-3 s  enable_temporal_fault=0  t_fault=1 s  enable_behavioral_fault=0  max_permissible_voltage_range=[-100, 100] V  t_fail_on_voltage=1 s  i_specify=off  i_priority=None  i=0 A  i_nominal_specify=off  i_nominal_unit=A  i_nominal_value=1  v_specify=off  v_priority=None  v=0 V  v_nominal_specify=off  v_nominal_unit=V  v_nominal_value=1  vc_specify=off  vc_priority=High  vc=0 V  vc_nominal_specify=off  vc_nominal_unit=V  vc_nominal_value=1
  Capacitor1 : ee_lib/Passive/Capacitor  cap_option=0  c=30e-6 F  Cvec=[1e-05, 1e-06] F  Vvec=[0, 10] V  CV_table_symmetry=1  f_vec=[1, 10] kHz  DFext_vec=[.8, 1.2]  enable_C_tol=0  C_tol=5  tol_distribution=1  nSigma=4  r=1e-6 Ohm  g=0 1/Ohm  averaging_period=0 s  enable_operating_limits=0  operating_limit_action=2  max_working_voltage_range=[-25, 25] V  power_rating=1 W  enable_faults=0  fault_action=1  Cscale_faulted=100  R_faulted=1e-3 Ohm  G_faulted=0 1/Ohm  tau_fault=1e-3 s  enable_temporal_fault=0  t_fault=1 s  enable_behavioral_fault=0  max_permissible_voltage_range=[-100, 100] V  t_fail_on_voltage=1 s  i_specify=off  i_priority=None  i=0 A  i_nominal_specify=off  i_nominal_unit=A  i_nominal_value=1  v_specify=off  v_priority=None  v=0 V  v_nominal_specify=off  v_nominal_unit=V  v_nominal_value=1  vc_specify=off  vc_priority=High  vc=0 V  vc_nominal_specify=off  vc_nominal_unit=V  vc_nominal_value=1
  Gate Driver{1..4} (4 alike) : ee_lib/Semiconductors & Converters/Gate Driver  uHighValue=0.7  uLowValue=0.3  vHigh=15 V  vLow=0 V  tHigh=T_on ns  tLow=T_off ns  parameterization=1  rHigh=R_on Ohm  rLow=R_off Ohm  tRise=20 ns  tFall=20 ns  cLoad=10 nF  enable_faults=0  t_fault=1 s  fault_type=1  ZonTime_specify=off  ZonTime_priority=None  ZonTime=0 s  ZoffTime_specify=off  ZoffTime_priority=None  ZoffTime=0 s  uHigh=2.0 V  uLow=0.8 V
      settings: SourceProductBaseCode=PS  InternalSimscapePortConfiguration="{\"Bottom\":[],\"Left\":[{\"id\":\"u\",\"label\":\"u\",\"type\":\"input\"}],\"Right\":[{\"id\":\"G\",\"label\":\"G\",\"type\":\"foundation.electrical.electrical\"},{\"id\":\"S\",\"label\":\"S\",\"type\":\"foundation.electrical.electrical\"}],\"Top\":[]}"
  S{1..4} (4 alike) : ee_lib/Semiconductors & Converters/IGBT (Ideal, Switching)  Vf=V_ft V  Ron=R_ont Ohm  Goff=1e-5 1/Ohm  Vth=6 V  diode_param=2  diode_Vf=V_fd V  diode_Ron=R_ond Ohm  diode_Goff=1e-5 1/Ohm  diode_C=50e-9 F  diode_iRM=-235 A  diode_iF=300 A  diode_idot=-50 A/us  diode_trr_param=ee.enum.converters.diodeReverseParam.trr_factor  diode_trr_factor=3  diode_trr=15 us  diode_Qrr=1500 s*uA  thermal_loss_option=ee.enum.converters.thermalLossOption.constantvalues  Von_data=[0, .1, .6, .8, 1, 1.3, 1.6, 2, 2.4; 0, .1, .7, 1, 1.2, 1.5, 1.9, 2.4, 2.8] V  Tj=[298.15, 398.15] K  Iout_data=[0, .1, 1, 5, 10, 20, 40, 70, 100] A  Eon_data=[0, .0024, .024, .12, .2, .48, 1.04, 2.16, 3.24; 0, .003, .03, .15, .25, .6, 1.3, 2.7, 4.05] * 1e-3 J  Eoff_data=[0, .0007, .0066, .033, .066, .17, .33, .83, 1.5; 0, .001, .01, .05, .1, .25, .5, 1.2, 2.2] * 1e-3 J  Tj_loss=[298.15, 398.15] K  Iout_data_loss=[0, .1, 1, 5, 10, 20, 40, 70, 100] A  Eon_scalar=22.86e-3 J  Eoff_scalar=17.14e-3 J  Voff=300 V  Iout_scalar=600 A  diodeModelType=ee.enum.converters.diodeModelType.pwl  diodeTableType=ee.enum.diode.tableType.IfMat  diode_IfMat=[.07, .12, .19, 1.75, 4.24, 7.32, 11.2; .16, .3, .72, 2.14, 4.02, 6.35, 9.12] A  diode_VfMat=[.9, 1.15, 1.25, 1.5, 1.75, 2.17, 2.6, 2.85; .58, .68, .75, 1.1, 1.38, 1.77, 2.27, 2.7] V  diode_TjVec=[25, 125] degC  diode_VfVec=[.5, .7, .9, 1.3, 1.7, 2.1, 2.5] V  diode_IfVec=[.1, .2, .5, 1, 2, 4, 7, 10] A  diode_Vr=-600 V  diode_Ls=150 nH  diode_Erec=0.03 J  thermal_network_parameterization=ee.enum.thermalNetworkTopology.external  Rth=[.08, .5] K/W  Rth_Cauer=[.08, .1, .5] K/W  Rth_Foster=[.08, .14, .22, .16] K/W  thermal_mass_parameterization=ee.enum.thermalNetwork.timeconstant  thermal_mass=[.01, .5] J/K  thermal_mass_Cauer=[.01, .1, .5] J/K  thermal_mass_Foster=[.001, .005, .05, .5] J/K  thermal_time_constant=[.001, .2] s  thermal_time_constant_Cauer=[.001, .1, .2] s  thermal_time_constant_Foster=[7e-05, .0007, .01, .08] s  thermal_mass_initial_temperatures=[25, 25] degC  thermal_mass_initial_temperatures_Cauer=[25, 25, 25] degC  junction_thermal_mass=0.01 J/K  steadyState_Foster=simscape.enum.onoff.on  Tvec_initial_Foster=[25, 25, 25, 25] degC  no_thermal_network=0  junction_temperature_specify=off  junction_temperature_priority=None  junction_temperature=25 degC  junction_temperature_nominal_specify=off  junction_temperature_nominal_unit=degC  junction_temperature_nominal_value=1  vT_specify=off  vT_priority=None  vT=0 V  vT_nominal_specify=off  vT_nominal_unit=V  vT_nominal_value=1  Qj_specify=off  Qj_priority=None  Qj=0 W  Qj_nominal_specify=off  Qj_nominal_unit=W  Qj_nominal_value=1
      settings: InternalSimscapePortConfiguration="{\"Bottom\":[],\"Left\":[{\"id\":\"G\",\"label\":\"\",\"type\":\"foundation.electrical.electrical\"}],\"Right\":[{\"id\":\"C\",\"label\":\"\",\"type\":\"foundation.electrical.electrical\"},{\"id\":\"E\",\"label\":\"\",\"type\":\"foundation.electrical.electrical\"}],\"Top\":[]}"
  vi : PMIOPort  Side=Right
  Q1 : PMIOPort  Port=2  Side=Left
  Q2 : PMIOPort  Port=3  Side=Left
  Q3 : PMIOPort  Port=4  Side=Left
  Q4 : PMIOPort  Port=5  Side=Left
  DC+ : PMIOPort  Port=6  Side=Left
  DC- : PMIOPort  Port=7  Side=Left
  GND : PMIOPort  Port=8  Side=Left
  connections:
  Capacitor1/RConn1 -- DC-/RConn1 -- Gate Driver3/RConn2 -- S4/RConn2
  S3/RConn1 -- vi/RConn1 -- S1/RConn2 -- Gate Driver4/RConn2 -- S4/RConn1
  GND/RConn1 -- Capacitor1/LConn1 -- Capacitor/RConn1 -- S2/RConn1
  Capacitor/LConn1 -- DC+/RConn1 -- S1/RConn1
  Gate Driver4/LConn1 -- Q1/RConn1
  Q3/RConn1 -- Gate Driver2/LConn1
  Gate Driver3/LConn1 -- Q4/RConn1
  S3/RConn2 -- Gate Driver1/RConn2 -- Gate Driver2/RConn2 -- S2/RConn2
  S1/LConn1 -- Gate Driver4/RConn1
  S4/LConn1 -- Gate Driver3/RConn1
  Gate Driver1/LConn1 -- Q2/RConn1
  S2/LConn1 -- Gate Driver1/RConn1
  S3/LConn1 -- Gate Driver2/RConn1

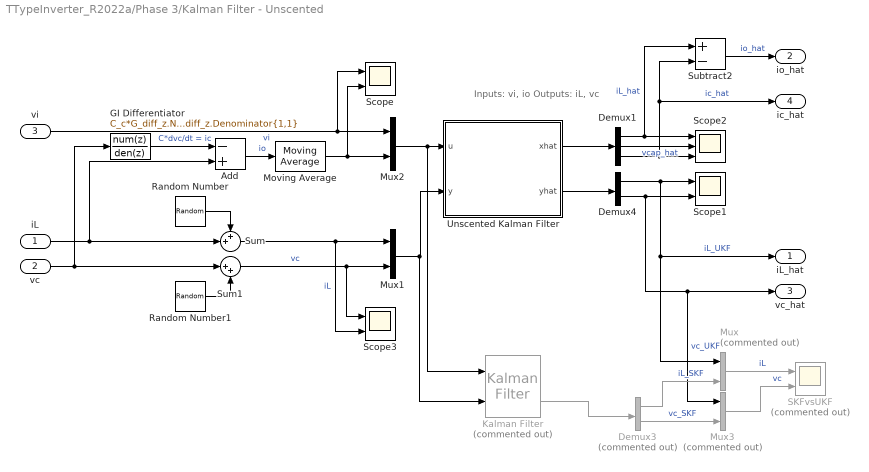
== system TTypeInverter_R2022a/Phase 3/Kalman Filter - Unscented ==
  note: Inputs: vi, io
      | Outputs: iL, vc
  iL : Inport
  vc : Inport  Port=2
  vi : Inport  Port=3
  Add : Sum  Inputs=-+
  Demux1 : Demux  Outputs=3
  Demux3 : Demux  Commented=on  Outputs=2
  Demux4 : Demux  Outputs=2
  GI Differentiator : DiscreteTransferFcn  Numerator=C_c*G_diff_z.Numerator{1,1}  Denominator=G_diff_z.Denominator{1,1}  SampleTime=Ts
  Kalman Filter : ctrlSharedLib/Kalman Filter  Commented=on  TimeDomain=Discrete-Time  UseCurrentEstimator=on  ModelSource=LTI State-Space Variable  ModelSourceVariable=lcl_sys_z  A=0.95  B=1  C=1  D=0  NumberOfStates=1  NumberOfInputs=1  NumberOfOutputs=1  InitialEstimateSource=Dialog  X0=0  P0=10  UseK=off  UseGH=off  NumberOfProcessNoiseInputs=1  G=1  TimeInvariantG=on  H=0  TimeInvariantH=on  Q=Q(1)  TimeInvariantQ=on  R=R  TimeInvariantR=on  N=N  TimeInvariantN=on  AddInputPort=on  AddEnablePort=off  OutputEstimatedY=on  OutputP=off  Ts=-1
  Moving Average : dspstat3/Moving Average  Method=Sliding window  ForgettingFactorPort=off  SpecifyWindowLength=on  WindowLength=4  ForgettingFactor=0.9  SimulateUsing=Code generation
  Mux : Mux  Commented=on  Inputs=2
  Mux1 : Mux  Inputs=2
  Mux2 : Mux  Inputs=2
  Mux3 : Mux  Commented=on  Inputs=2
  Random Number : RandomNumber  Variance=R(1,1)  SampleTime=Ts
  Random Number1 : RandomNumber  Variance=R(2,2)  SampleTime=Ts
  SKFvsUKF : Scope  Commented=on  NumInputPorts=2
  Scope : Scope  NumInputPorts=2
  Scope1 : Scope  NumInputPorts=2
  Scope2 : Scope  NumInputPorts=3
  Scope3 : Scope  NumInputPorts=2
  Subtract2 : Sum  Inputs=+-
  Sum : Sum  Inputs=++|
  Sum1 : Sum  Inputs=|++
  Unscented Kalman Filter : Subsystem
  iL_hat : Outport
  io_hat : Outport  Port=2
  vc_hat : Outport  Port=3
  ic_hat : Outport  Port=4
  wires:
  Demux4/1 -> Mux/1, iL_hat/1, Scope1/1  "iL_UKF"
  Demux1/2 -> Scope2/2  "vcap_hat"
  Demux1/3 -> ic_hat/1, Subtract2/2, Scope2/3  "ic_hat"
  Demux1/1 -> Subtract2/1, Scope2/1  "iL_hat"
  Mux1/1 -> Kalman Filter/2, Unscented Kalman Filter/2(y)
  GI Differentiator/1 -> Add/1  "C*dvc/dt = ic"
  vi/1 -> Scope/1, Mux2/1  "vi"
  Demux4/2 -> Scope1/2, Mux3/1, vc_hat/1  "vc_UKF"
  Unscented Kalman Filter/2(yhat) -> Demux4/1
  vc/1 -> Sum1/1, GI Differentiator/1
  Unscented Kalman Filter/1(xhat) -> Demux1/1
  iL/1 -> Sum/2, Add/2
  Sum/1 -> Scope3/2, Mux1/1  "iL"
  Sum1/1 -> Scope3/1, Mux1/2  "vc"
  Random Number/1 -> Sum/1
  Random Number1/1 -> Sum1/2
  Mux2/1 -> Kalman Filter/1, Unscented Kalman Filter/1(u)
  Subtract2/1 -> io_hat/1  "io_hat"
  Add/1 -> Moving Average/1  "io"
  Moving Average/1 -> Mux2/2, Scope/2
  Kalman Filter/2 -> Demux3/1
  Mux/1 -> SKFvsUKF/1  "iL"
  Demux3/1 -> Mux/2  "iL_SKF"
  Mux3/1 -> SKFvsUKF/2  "vc"
  Demux3/2 -> Mux3/2  "vc_SKF"

== system TTypeInverter_R2022a/Phase 3/Output Filter ==
  Cc : ee_lib/Passive/Capacitor  cap_option=0  c=C_c F  Cvec=[1e-05, 1e-06] F  Vvec=[0, 10] V  CV_table_symmetry=1  f_vec=[1, 10] kHz  DFext_vec=[.8, 1.2]  enable_C_tol=0  C_tol=5  tol_distribution=1  nSigma=4  r=R_Cc Ohm  g=0 1/Ohm  averaging_period=0 s  enable_operating_limits=0  operating_limit_action=2  max_working_voltage_range=[-25, 25] V  power_rating=1 W  enable_faults=0  fault_action=1  Cscale_faulted=100  R_faulted=1e-3 Ohm  G_faulted=0 1/Ohm  tau_fault=1e-3 s  enable_temporal_fault=0  t_fault=1 s  enable_behavioral_fault=0  max_permissible_voltage_range=[-100, 100] V  t_fail_on_voltage=1 s  i_specify=off  i_priority=None  i=0 A  i_nominal_specify=off  i_nominal_unit=A  i_nominal_value=1  v_specify=off  v_priority=None  v=0 V  v_nominal_specify=off  v_nominal_unit=V  v_nominal_value=1  vc_specify=off  vc_priority=High  vc=-280 V  vc_nominal_specify=off  vc_nominal_unit=V  vc_nominal_value=1
  Cr : ee_lib/Passive/Capacitor  cap_option=0  c=C_r F  Cvec=[1e-05, 1e-06] F  Vvec=[0, 10] V  CV_table_symmetry=1  f_vec=[1, 10] kHz  DFext_vec=[.8, 1.2]  enable_C_tol=0  C_tol=5  tol_distribution=1  nSigma=4  r=R_Cr Ohm  g=0 1/Ohm  averaging_period=0 s  enable_operating_limits=0  operating_limit_action=2  max_working_voltage_range=[-25, 25] V  power_rating=1 W  enable_faults=0  fault_action=1  Cscale_faulted=100  R_faulted=1e-3 Ohm  G_faulted=0 1/Ohm  tau_fault=1e-3 s  enable_temporal_fault=0  t_fault=1 s  enable_behavioral_fault=0  max_permissible_voltage_range=[-100, 100] V  t_fail_on_voltage=1 s  i_specify=off  i_priority=None  i=0 A  i_nominal_specify=off  i_nominal_unit=A  i_nominal_value=1  v_specify=off  v_priority=None  v=0 V  v_nominal_specify=off  v_nominal_unit=V  v_nominal_value=1  vc_specify=off  vc_priority=High  vc=0 V  vc_nominal_specify=off  vc_nominal_unit=V  vc_nominal_value=1
  Current Sensor : fl_lib/Electrical/Electrical Sensors/Current Sensor
      settings: SourceProductBaseCode=PW,SS,VE
  Current Sensor2 : fl_lib/Electrical/Electrical Sensors/Current Sensor
      settings: SourceProductBaseCode=PW,SS,VE
  Electrical Reference1 : fl_lib/Electrical/Electrical Elements/Electrical Reference
      settings: SourceProductBaseCode=PW,SS,VE
  Lc : ee_lib/Passive/Inductor  l=L_c H  enable_L_tol=0  L_tol=20  tol_distribution=1  nSigma=4  r=R_Lc Ohm  g=1e-9 1/Ohm  enable_operating_limits=0  operating_limit_action=2  max_working_current=1 A  power_rating=1 W  enable_faults=0  fault_action=1  lambdaPercent=50  k_faulted=0.9999  turnsShort=0  openCct=0  groundShort=0  groundShortG=0 1/Ohm  tau_fault=1e-3 s  enable_temporal_fault=0  t_fault=1 s  enable_behavioral_fault=0  max_permissible_voltage=100 V  n_fail_on_voltage=1  max_permissible_current=1 A  t_fail_on_current=1 s  i_L_specify=off  i_L_priority=High  i_L=0 A  i_L_nominal_specify=off  i_L_nominal_unit=A  i_L_nominal_value=1
  "Lc (Nonlinear, phi-I)" : ee_lib/Passive/Nonlinear Inductor  parameterization_option=3  Nw=N_Lc  L=2e-4 H  L_sat=1e-4 H  current_data=Lc_nonlin_i A  magnetic_flux_data=Lc_nonlin_phi Wb  H_data=[0, 200, 400, 600, 800, 1000] A/m  B_data=[0, .81, 1.25, 1.42, 1.48, 1.49] T  magnetic_flux_sat=1.3e-05 Wb  length_effective=0.032 m  area_effective=1.6e-5 m^2  dBdH0=0.005 T*m/A  B1=1.49 T  H1=1000 A/m  c=0.1  K=200 A/m  alpha=1e-4  averaging_period=0 s  G_parasitic=1e-9 1/Ohm  interpolation_option=1  x0_option=1  i_L0=0 A  phi0=0 Wb  B0=0 T  H0=0 A/m
      settings: SourceProductBaseCode=PS  InternalSimscapePortConfiguration="{\"Bottom\":[],\"Left\":[{\"id\":\"p\",\"label\":\"+\",\"type\":\"foundation.electrical.electrical\"}],\"Right\":[{\"id\":\"n\",\"label\":\"-\",\"type\":\"foundation.electrical.electrical\"}],\"Top\":[]}"
  Lg : ee_lib/Passive/Inductor  l=L_g H  enable_L_tol=0  L_tol=20  tol_distribution=1  nSigma=4  r=R_Lg Ohm  g=1e-9 1/Ohm  enable_operating_limits=0  operating_limit_action=2  max_working_current=1 A  power_rating=1 W  enable_faults=0  fault_action=1  lambdaPercent=50  k_faulted=0.9999  turnsShort=0  openCct=0  groundShort=0  groundShortG=0 1/Ohm  tau_fault=1e-3 s  enable_temporal_fault=0  t_fault=1 s  enable_behavioral_fault=0  max_permissible_voltage=100 V  n_fail_on_voltage=1  max_permissible_current=1 A  t_fail_on_current=1 s  i_L_specify=off  i_L_priority=High  i_L=0 A  i_L_nominal_specify=off  i_L_nominal_unit=A  i_L_nominal_value=1
  Lr : ee_lib/Passive/Inductor  l=L_r H  enable_L_tol=0  L_tol=20  tol_distribution=1  nSigma=4  r=R_Lr Ohm  g=1e-9 1/Ohm  enable_operating_limits=0  operating_limit_action=2  max_working_current=1 A  power_rating=1 W  enable_faults=0  fault_action=1  lambdaPercent=50  k_faulted=0.9999  turnsShort=0  openCct=0  groundShort=0  groundShortG=0 1/Ohm  tau_fault=1e-3 s  enable_temporal_fault=0  t_fault=1 s  enable_behavioral_fault=0  max_permissible_voltage=100 V  n_fail_on_voltage=1  max_permissible_current=1 A  t_fail_on_current=1 s  i_L_specify=off  i_L_priority=High  i_L=0 A  i_L_nominal_specify=off  i_L_nominal_unit=A  i_L_nominal_value=1
  RLc : fl_lib/Electrical/Electrical Elements/Resistor  R=R_Lc Ohm  i_specify=off  i_priority=None  i=0 A  i_nominal_specify=off  i_nominal_unit=A  i_nominal_value=1  v_specify=off  v_priority=None  v=0 V  v_nominal_specify=off  v_nominal_unit=V  v_nominal_value=1
      settings: SourceProductBaseCode=PW,SS,VE
  Voltage Sensor : fl_lib/Electrical/Electrical Sensors/Voltage Sensor
      settings: SourceProductBaseCode=PW,SS,VE
  vi : PMIOPort  Side=Left
  vo : PMIOPort  Port=2  Side=Right
  GND : PMIOPort  Port=3  Side=Right
  ic : PMIOPort  Port=4  Side=Right
  vc : PMIOPort  Port=5  Side=Right
  iL : PMIOPort  Port=6  Side=Right
  connections:
  Lr/LConn1 -- Cr/RConn1
  Voltage Sensor/RConn1 -- vc/RConn1
  Current Sensor/LConn1 -- vi/RConn1
  Electrical Reference1/LConn1 -- Voltage Sensor/RConn2 -- Cc/RConn1 -- Lr/RConn1 -- GND/RConn1
  Lg/RConn1 -- vo/RConn1
  Voltage Sensor/LConn1 -- Current Sensor2/LConn1 -- Lg/LConn1 -- Cr/LConn1 -- RLc/RConn1
  "Lc (Nonlinear, phi-I)"/LConn1 -- Current Sensor/RConn2
  Current Sensor/RConn1 -- iL/RConn1
  Current Sensor2/RConn2 -- Cc/LConn1
  Current Sensor2/RConn1 -- ic/RConn1
  "Lc (Nonlinear, phi-I)"/RConn1 -- RLc/LConn1

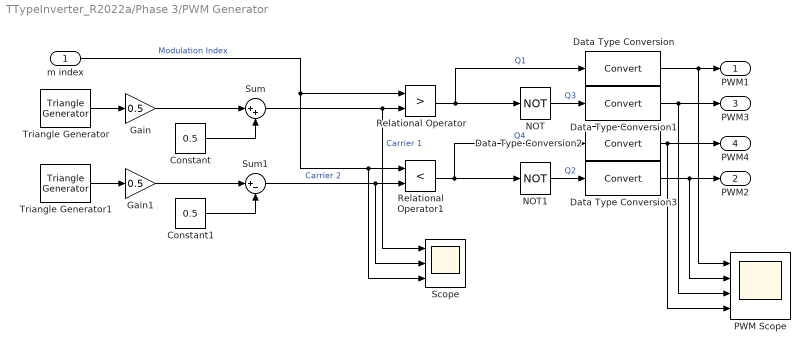
== system TTypeInverter_R2022a/Phase 3/PWM Generator ==
  m index : Inport
  Constant : Constant  Value=0.5
  Constant1 : Constant  Value=0.5
  Data Type Conversion{,1..3} (4 alike) : DataTypeConversion  SaturateOnIntegerOverflow=off  RndMeth=Floor
  Gain : Gain  Gain=0.5
  Gain1 : Gain  Gain=0.5
  NOT : Logic  Operator=NOT  IconShape=distinctive  AllPortsSameDT=off  OutDataTypeStr=boolean
  NOT1 : Logic  Operator=NOT  IconShape=distinctive  AllPortsSameDT=off  OutDataTypeStr=boolean
  PWM Scope : Scope  NumInputPorts=4
  Relational Operator : RelationalOperator  Operator=>  OutDataTypeStr=boolean  RndMeth=Simplest  InputSameDT=off
  Relational Operator1 : RelationalOperator  Operator=<  OutDataTypeStr=boolean  RndMeth=Simplest  InputSameDT=off
  Scope : Scope  NumInputPorts=3
  Sum : Sum  Inputs=|++
  Sum1 : Sum  Inputs=|+-
  Triangle Generator : spsTriangleGeneratorLib/Triangle Generator  Freq=f_sw  Phase=0  Ts=0
  Triangle Generator1 : spsTriangleGeneratorLib/Triangle Generator  Freq=f_sw  Phase=0  Ts=0
  PWM1 : Outport
  PWM2 : Outport  Port=2
  PWM3 : Outport  Port=3
  PWM4 : Outport  Port=4
  wires:
  Relational Operator1/1 -> NOT1/1, Data Type Conversion2/1  "Q4"
  Data Type Conversion3/1 -> PWM2/1, PWM Scope/2
  Constant/1 -> Sum/2
  Gain/1 -> Sum/1
  NOT1/1 -> Data Type Conversion3/1  "Q2"
  NOT/1 -> Data Type Conversion1/1  "Q3"
  m index/1 -> Scope/3, Relational Operator1/1, Relational Operator/1  "Modulation Index"
  Data Type Conversion2/1 -> PWM4/1, PWM Scope/4
  Data Type Conversion1/1 -> PWM3/1, PWM Scope/3
  Triangle Generator1/1 -> Gain1/1
  Relational Operator/1 -> Data Type Conversion/1, NOT/1  "Q1"
  Data Type Conversion/1 -> PWM1/1, PWM Scope/1
  Triangle Generator/1 -> Gain/1
  Sum1/1 -> Scope/2, Relational Operator1/2  "Carrier 2"
  Sum/1 -> Scope/1, Relational Operator/2  "Carrier 1"
  Constant1/1 -> Sum1/2
  Gain1/1 -> Sum1/1
